simulink model "PumpCalibration"  (R2019a)
settings: Solver=FixedStepAuto  StartTime=0.0  StopTime=inf  RelTol=1e-3
settings Model: EnablePacing=on  Creator=wuyua  LastModifiedBy=wuyua
settings DataIOCC: ReturnWorkspaceOutputs=off
settings DebuggingCC: ArithmeticOperatorsInVariantConditions=warning

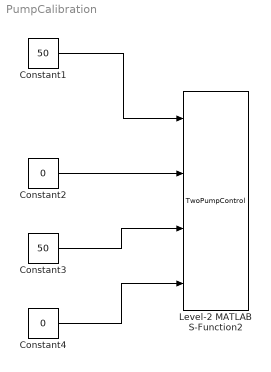
== system PumpCalibration ==
  Constant1 : Constant  Value=50  OutDataTypeStr=single
  Constant2 : Constant  Value=0  OutDataTypeStr=int8
  Constant3 : Constant  Value=50  OutDataTypeStr=single
  Constant4 : Constant  Value=0  OutDataTypeStr=int8
  Level-2 MATLAB S-Function2 : M-S-Function  FunctionName=TwoPumpControl
  wires:
  Constant1/1 -> Level-2 MATLAB S-Function2/1
  Constant2/1 -> Level-2 MATLAB S-Function2/2
  Constant3/1 -> Level-2 MATLAB S-Function2/3
  Constant4/1 -> Level-2 MATLAB S-Function2/4
